simulink model "SegOrdemZero"  (R2015a)
settings: Solver=ode45  StartTime=0.0  StopTime=50  FixedStep=0.00001
settings Model: Creator=user  LastModifiedBy=user
settings SolverCC: ShapePreserveControl=EnableAll  ZeroCrossAlgorithm=Adaptive
settings DebuggingCC: UnderspecifiedInitializationDetection=Classic

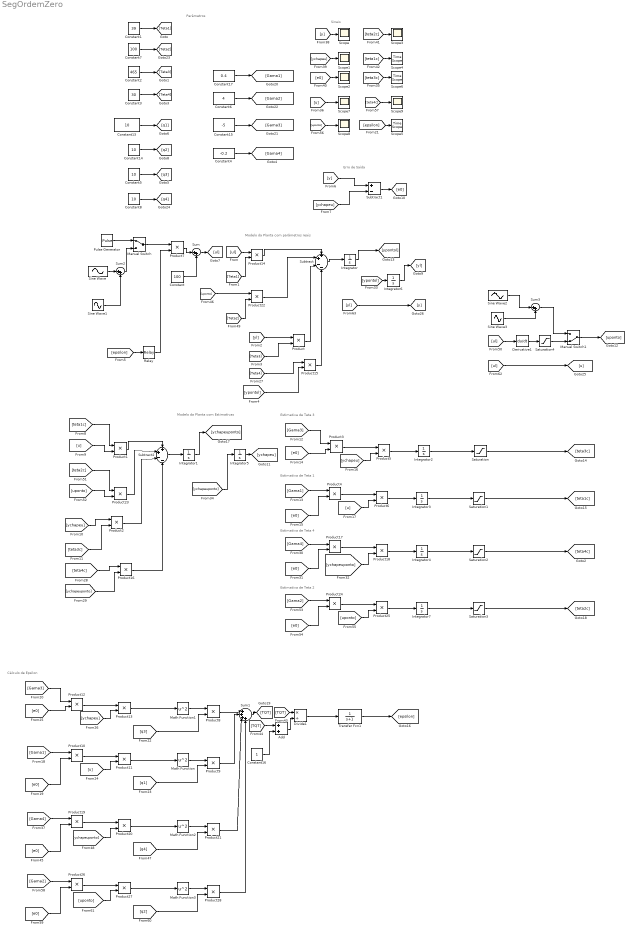
== system SegOrdemZero ==
  note: Cálculo de Epsilon
  note: Estimativa de Teta 1
  note: Estimativa de Teta 3
  note: Modelo da Planta com Estimativas
  note: Modelo da Planta com parâmetros reais
  note: Erro de Saída
  note: Parâmetros
  note: Sinais
  note: Estimativa de Teta 4
  note: Estimativa de Teta 2
  Add : Sum  AccumDataTypeStr=double
  Constant : Constant  Value=100
  Constant1 : Constant  Value=39
  Constant{5,8,13..14} (4 alike) : Constant  Value=10
  Constant15 : Constant  Value=-5
  Constant16 : Constant
  Constant17 : Constant  Value=0.4
  Constant2 : Constant  Value=465
  Constant3 : Constant  Value=30
  Constant4 : Constant  Value=-0.2
  Constant6 : Constant  Value=4
  Constant7 : Constant  Value=100
  Derivative1 : Derivative
  Divide1 : Product  Inputs=*/  OutDataTypeStr=double
  Integrator{,1,5..6} (4 alike) : Integrator
  Integrator2 : Integrator  InitialCondition=70
  Integrator3 : Integrator  InitialCondition=80
  Integrator4 : Integrator  InitialCondition=5
  Integrator7 : Integrator  InitialCondition=98
  Manual Switch : ManualSwitch
  Manual Switch1 : ManualSwitch  CurrentSetting=0
  Math Function{,1..3} (4 alike) : Math  Operator=square  SaturateOnIntegerOverflow=on
  Product{,1..28} (29 alike) : Product
  Pulse Generator : DiscretePulseGenerator  PulseType=Time based  Amplitude=100  Period=1  PulseWidth=50
  Relay : Relay  OnSwitchValue=0.5  OffSwitchValue=0.05
  Saturation : Saturate  UpperLimit=50000  LowerLimit=0
  Saturation1 : Saturate  UpperLimit=300000  LowerLimit=1
  Saturation2 : Saturate  UpperLimit=30000  LowerLimit=0
  Saturation3 : Saturate  UpperLimit=300000  LowerLimit=1
  Saturation4 : Saturate  UpperLimit=165  LowerLimit=-165
  Scope{,1..3,7..9} (7 alike) : Scope
      Scope settings: YMin=-20  YMax=45
      Scope1 settings: YMin=-20  YMax=45  SampleInput=on
      Scope2 settings: YMin=-0.012  YMax=0.012  SaveName=ScopeData2  SampleInput=on
      Scope3 settings: TimeRange=125  YMin=331  YMax=340  SaveName=ScopeData3  SampleInput=on
      Scope7 settings: YMin=95  YMax=105  SaveName=ScopeData5  SampleInput=on
      Scope8 settings: YMin=-125  YMax=150  SaveName=ScopeData4  SampleInput=on
      Scope9 settings: YMin=40  YMax=95  SaveName=ScopeData6  SampleInput=on
  Scope4 : TimeScope
  Scope5 : TimeScope
  Scope6 : TimeScope
  Sine Wave : Sin  Amplitude=50  SampleTime=0
  Sine Wave1 : Sin  Amplitude=50  Frequency=2  SampleTime=0
  Sine Wave2 : Sin  Amplitude=50  Phase=pi/2  SampleTime=0
  Sine Wave3 : Sin  Amplitude=100  Frequency=2  Phase=pi/2  SampleTime=0
  Subtract : Sum  Inputs=++--
  Subtract1 : Sum  Inputs=+-
  Subtract2 : Sum  Inputs=++--
  Sum : Sum  Inputs=|++
  Sum1 : Sum  Inputs=|++++
  Sum2 : Sum  Inputs=|++
  Sum3 : Sum  Inputs=|++
  Transfer Fcn1 : TransferFcn  Denominator=[1 1]
  wires:
  Constant/1 -> Sum/2
  [Teta1] -> Product14/2
  [Teta3] -> Product/2
  Product14/1 -> Subtract/1
  Subtract/1 -> Integrator/1
  [yl] -> Product/1
  Sum/1 -> [ul]
  [ul] -> Product14/1
  [y] -> Subtract1/1
  [ychapeu] -> Subtract1/2
  Subtract1/1 -> [e0]
  Constant1/1 -> [Teta1]
  Constant2/1 -> [Teta3]
  Product1/1 -> Subtract2/1
  Subtract2/1 -> Integrator1/1
  [teta3c] -> Product2/2
  [ychapeu] -> Product2/1
  [u] -> Product1/2
  [teta1c] -> Product1/1
  [e0] -> Product3/2
  [Gama3] -> Product3/1
  [Gama1] -> Product4/1
  [e0] -> Product4/2
  Product4/1 -> Product6/1
  Product3/1 -> Product5/1
  [ychapeu] -> Product5/2
  [u] -> Product6/2
  Product5/1 -> Integrator2/1
  Product6/1 -> Integrator3/1
  Integrator2/1 -> Saturation/1
  Product7/1 -> Sum/1
  Product11/1 -> Math Function/1
  Product13/1 -> Math Function1/1
  Math Function1/1 -> Product8/1
  Math Function/1 -> Product9/1
  [q3] -> Product8/2
  [q1] -> Product9/2
  Product9/1 -> Sum1/2
  Product8/1 -> Sum1/1
  Constant13/1 -> [q1]
  Constant14/1 -> [q2]
  [y] -> Scope/1
  [ychapeu] -> Scope1/1
  [e0] -> Scope2/1
  [teta2c] -> Scope3/1
  [teta1c] -> Scope4/1
  Constant17/1 -> [Gama1]
  Constant15/1 -> [Gama3]
  Add/1 -> Divide1/2
  Constant16/1 -> Add/2
  Sum1/1 -> [TQT]
  [TQT] -> Divide1/1
  [TQT] -> Add/1
  [epsilon] -> Relay/1
  Saturation/1 -> [teta3c]
  Saturation1/1 -> [teta1c]
  [Gama1] -> Product10/1
  [e0] -> Product10/2
  Product10/1 -> Product11/1
  [u] -> Product11/2
  [e0] -> Product12/2
  [Gama3] -> Product12/1
  Product12/1 -> Product13/1
  [ychapeu] -> Product13/2
  Relay/1 -> Product7/2
  [epsilon] -> Scope5/1
  [ypontol] -> Product15/2
  [Teta4] -> Product15/1
  [ychapeuponto] -> Product16/2
  [teta4c] -> Product16/1
  [Gama4] -> Product17/1
  [e0] -> Product17/2
  Product17/1 -> Product18/1
  [ychapeuponto] -> Product18/2
  Product18/1 -> Integrator4/1
  Integrator4/1 -> Saturation2/1
  Saturation2/1 -> [teta4c]
  Constant3/1 -> [Teta4]
  Constant4/1 -> [Gama4]
  Constant5/1 -> [q3]
  Integrator5/1 -> [ychapeu]
  Integrator6/1 -> [yl]
  Integrator/1 -> [ypontol]
  [ypontol] -> Integrator6/1
  [ychapeuponto] -> Integrator5/1
  Integrator1/1 -> [ychapeuponto]
  [teta3c] -> Scope6/1
  Divide1/1 -> Transfer Fcn1/1
  [u] -> Scope7/1
  Product20/1 -> Math Function2/1
  Math Function2/1 -> Product21/1
  [q4] -> Product21/2
  [Gama4] -> Product19/1
  [e0] -> Product19/2
  Product19/1 -> Product20/1
  [ychapeuponto] -> Product20/2
  Product21/1 -> Sum1/3
  Product15/1 -> Subtract/4
  Product/1 -> Subtract/3
  [Teta2] -> Product22/2
  [uponto] -> Product22/1
  Product22/1 -> Subtract/2
  Product16/1 -> Subtract2/4
  Product2/1 -> Subtract2/3
  [uponto] -> Product23/2
  [teta2c] -> Product23/1
  Product23/1 -> Subtract2/2
  [Gama2] -> Product24/1
  [e0] -> Product24/2
  Product24/1 -> Product25/1
  [uponto] -> Product25/2
  Product25/1 -> Integrator7/1
  Integrator7/1 -> Saturation3/1
  Saturation3/1 -> [teta2c]
  Constant6/1 -> [Gama2]
  Constant7/1 -> [Teta2]
  Constant8/1 -> [q4]
  [uponto] -> Scope8/1
  [teta4c] -> Scope9/1
  Product27/1 -> Math Function3/1
  Math Function3/1 -> Product28/1
  [q2] -> Product28/2
  [Gama2] -> Product26/1
  [e0] -> Product26/2
  Product26/1 -> Product27/1
  [uponto] -> Product27/2
  Product28/1 -> Sum1/4
  [ul] -> Derivative1/1
  Transfer Fcn1/1 -> [epsilon]
  [ul] -> [u]
  [yl] -> [y]
  Derivative1/1 -> Saturation4/1
  Pulse Generator/1 -> Manual Switch/1
  Manual Switch/1 -> Product7/1
  Sine Wave/1 -> Sum2/1
  Sine Wave1/1 -> Sum2/2
  Sum2/1 -> Manual Switch/2
  Integrator3/1 -> Saturation1/1
  Manual Switch1/1 -> [uponto]
  Saturation4/1 -> Manual Switch1/2
  Sine Wave3/1 -> Sum3/2
  Sine Wave2/1 -> Sum3/1
  Sum3/1 -> Manual Switch1/1
